simulink model "TorqueAllocator"  (R2026b)
settings: Solver=FixedStepDiscrete  StopTime=0.1  FixedStep=UnifiedControlSampleTime
settings Model: DataDictionary=VehicleData.sldd  Creator=Xu Dingyi  LastModifiedBy=29358

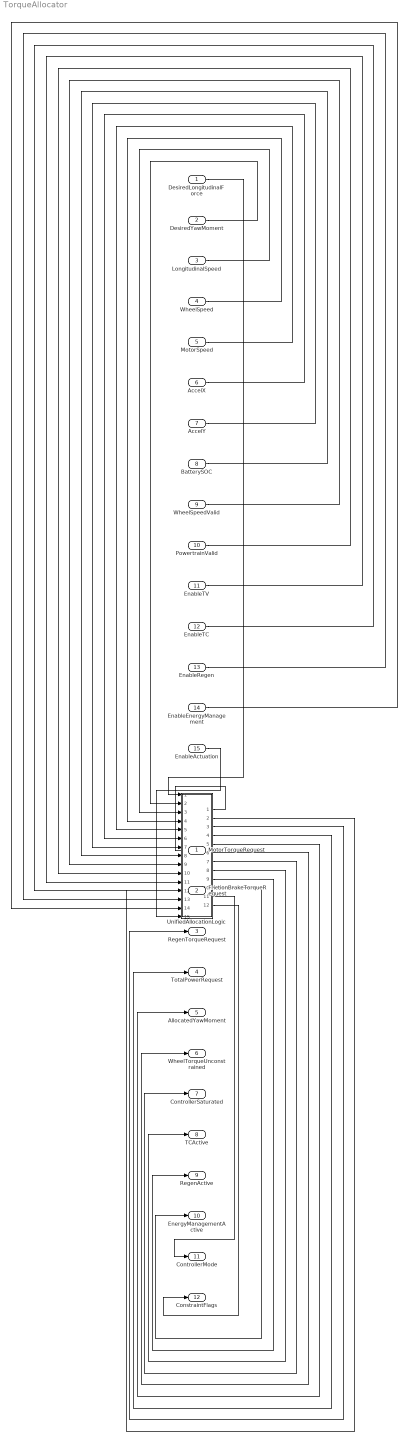
== system TorqueAllocator ==
  DesiredLongitudinalForce : Inport  OutDataTypeStr=double  PortDimensions=1
  DesiredYawMoment : Inport  Port=2  OutDataTypeStr=double  PortDimensions=1
  LongitudinalSpeed : Inport  Port=3  OutDataTypeStr=double  PortDimensions=1
  WheelSpeed : Inport  Port=4  OutDataTypeStr=double  PortDimensions=4
  MotorSpeed : Inport  Port=5  OutDataTypeStr=double  PortDimensions=4
  AccelX : Inport  Port=6  OutDataTypeStr=double  PortDimensions=1
  AccelY : Inport  Port=7  OutDataTypeStr=double  PortDimensions=1
  BatterySOC : Inport  Port=8  OutDataTypeStr=double  PortDimensions=1
  WheelSpeedValid : Inport  Port=9  OutDataTypeStr=boolean  PortDimensions=4
  PowertrainValid : Inport  Port=10  OutDataTypeStr=boolean  PortDimensions=1
  EnableTV : Inport  Port=11  OutDataTypeStr=boolean  PortDimensions=1
  EnableTC : Inport  Port=12  OutDataTypeStr=boolean  PortDimensions=1
  EnableRegen : Inport  Port=13  OutDataTypeStr=boolean  PortDimensions=1
  EnableEnergyManagement : Inport  Port=14  OutDataTypeStr=boolean  PortDimensions=1
  EnableActuation : Inport  Port=15  OutDataTypeStr=boolean  PortDimensions=1
  UnifiedAllocationLogic : Stateflow chart  TreatAsAtomicUnit=on
  MotorTorqueRequest : Outport  OutDataTypeStr=double  PortDimensions=4
  FrictionBrakeTorqueRequest : Outport  Port=2  OutDataTypeStr=double  PortDimensions=4
  RegenTorqueRequest : Outport  Port=3  OutDataTypeStr=double  PortDimensions=4
  TotalPowerRequest : Outport  Port=4  OutDataTypeStr=double  PortDimensions=1
  AllocatedYawMoment : Outport  Port=5  OutDataTypeStr=double  PortDimensions=1
  WheelTorqueUnconstrained : Outport  Port=6  OutDataTypeStr=double  PortDimensions=4
  ControllerSaturated : Outport  Port=7  OutDataTypeStr=boolean  PortDimensions=1
  TCActive : Outport  Port=8  OutDataTypeStr=boolean  PortDimensions=1
  RegenActive : Outport  Port=9  OutDataTypeStr=boolean  PortDimensions=1
  EnergyManagementActive : Outport  Port=10  OutDataTypeStr=boolean  PortDimensions=1
  ControllerMode : Outport  Port=11  OutDataTypeStr=uint8  PortDimensions=1
  ConstraintFlags : Outport  Port=12  OutDataTypeStr=uint16  PortDimensions=1
  wires:
  DesiredLongitudinalForce/1 -> UnifiedAllocationLogic/1(DesiredLongitudinalForce)
  DesiredYawMoment/1 -> UnifiedAllocationLogic/2(DesiredYawMoment)
  LongitudinalSpeed/1 -> UnifiedAllocationLogic/3(LongitudinalSpeed)
  WheelSpeed/1 -> UnifiedAllocationLogic/4(WheelSpeed)
  MotorSpeed/1 -> UnifiedAllocationLogic/5(MotorSpeed)
  AccelX/1 -> UnifiedAllocationLogic/6(AccelX)
  AccelY/1 -> UnifiedAllocationLogic/7(AccelY)
  BatterySOC/1 -> UnifiedAllocationLogic/8(BatterySOC)
  WheelSpeedValid/1 -> UnifiedAllocationLogic/9(WheelSpeedValid)
  PowertrainValid/1 -> UnifiedAllocationLogic/10(PowertrainValid)
  EnableTV/1 -> UnifiedAllocationLogic/11(EnableTV)
  EnableTC/1 -> UnifiedAllocationLogic/12(EnableTC)
  EnableRegen/1 -> UnifiedAllocationLogic/13(EnableRegen)
  EnableEnergyManagement/1 -> UnifiedAllocationLogic/14(EnableEnergyManagement)
  EnableActuation/1 -> UnifiedAllocationLogic/15(EnableActuation)
  UnifiedAllocationLogic/1(MotorTorqueRequest) -> MotorTorqueRequest/1
  UnifiedAllocationLogic/2(FrictionBrakeTorqueRequest) -> FrictionBrakeTorqueRequest/1
  UnifiedAllocationLogic/3(RegenTorqueRequest) -> RegenTorqueRequest/1
  UnifiedAllocationLogic/4(TotalPowerRequest) -> TotalPowerRequest/1
  UnifiedAllocationLogic/5(AllocatedYawMoment) -> AllocatedYawMoment/1
  UnifiedAllocationLogic/6(WheelTorqueUnconstrained) -> WheelTorqueUnconstrained/1
  UnifiedAllocationLogic/7(ControllerSaturated) -> ControllerSaturated/1
  UnifiedAllocationLogic/8(TCActive) -> TCActive/1
  UnifiedAllocationLogic/9(RegenActive) -> RegenActive/1
  UnifiedAllocationLogic/10(EnergyManagementActive) -> EnergyManagementActive/1
  UnifiedAllocationLogic/11(ControllerMode) -> ControllerMode/1
  UnifiedAllocationLogic/12(ConstraintFlags) -> ConstraintFlags/1

== stateflow chart TorqueAllocator/UnifiedAllocationLogic ==
  state Allocate
    en: PreviousMotorTorque = zeros(4,1); TCState = false(4,1);
    du: [MotorTorqueRequest, FrictionBrakeTorqueRequest, RegenTorqueRequest, TotalPowerRequest, AllocatedYawMoment, WheelTorqueUnconstrained, ControllerSaturated, TCActive, RegenActive, EnergyManagementActive, ControllerMode, ConstraintFlags, PreviousMotorTorque, TCState] = unifiedControlUnifiedAllocationStep(DesiredLongitudinalForce, DesiredYawMoment, LongitudinalSpeed, WheelSpeed, MotorSpeed, AccelX, AccelY, BatterySOC, WheelSpeedValid, PowertrainValid, EnableTV, EnableTC, EnableRegen, EnableEnergyManagement, EnableActuation, PreviousMotorTorque, TCState, UnifiedControlSampleTime, UnifiedControlVehicleMass, UnifiedControlGravity, UnifiedControlWheelbase, UnifiedControlCGHeight, UnifiedControlStaticLoadDistributionFront, UnifiedControlRollStiffnessDistributionFront, UnifiedControlTrackFront, UnifiedControlTrackRear, UnifiedControlTireEffectiveRadius, UnifiedControlLowSpeedEpsilon, UnifiedControlGearRatio, UnifiedControlGearEfficiency, UnifiedControlMotorTorqueLimit, UnifiedControlMotorSpeedLimit, UnifiedControlInverterEfficiency, UnifiedControlDrivePowerLimit, UnifiedControlRegenPowerLimit, UnifiedControlBrakeMaxTorque, UnifiedControlBatterySOCUpperLimit, UnifiedControlPowerEpsilon, UnifiedControlMotorTorqueRateLimit, UnifiedControlFrictionEstimate, UnifiedControlTCSlipOn, UnifiedControlTCSlipOff, UnifiedControlTCSlipFullCut, UnifiedControlMinimumNormalLoad, UnifiedControlEnergyDriveFraction, UnifiedControlForcePriorityWeight, UnifiedControlYawPriorityWeight, UnifiedControlRegularizationWeight, UnifiedControlAllocatorIterations);
  (default) -> Allocate
  data: DesiredLongitudinalForce input double; DesiredYawMoment input double; LongitudinalSpeed input double; WheelSpeed input double; MotorSpeed input double; AccelX input double; AccelY input double; BatterySOC input double; WheelSpeedValid input boolean; PowertrainValid input boolean; EnableTV input boolean; EnableTC input boolean; EnableRegen input boolean; EnableEnergyManagement input boolean; EnableActuation input boolean; MotorTorqueRequest output double; FrictionBrakeTorqueRequest output double; RegenTorqueRequest output double; TotalPowerRequest output double; AllocatedYawMoment output double; WheelTorqueUnconstrained output double; ControllerSaturated output boolean; TCActive output boolean; RegenActive output boolean; EnergyManagementActive output boolean; ControllerMode output uint8; ConstraintFlags output uint16; PreviousMotorTorque local double; TCState local boolean; UnifiedControlSampleTime parameter double; UnifiedControlVehicleMass parameter double; UnifiedControlGravity parameter double; UnifiedControlWheelbase parameter double; UnifiedControlCGHeight parameter double; UnifiedControlStaticLoadDistributionFront parameter double; UnifiedControlRollStiffnessDistributionFront parameter double; UnifiedControlTrackFront parameter double; UnifiedControlTrackRear parameter double; UnifiedControlTireEffectiveRadius parameter double; UnifiedControlLowSpeedEpsilon parameter double; UnifiedControlGearRatio parameter double; UnifiedControlGearEfficiency parameter double; UnifiedControlMotorTorqueLimit parameter double; UnifiedControlMotorSpeedLimit parameter double; UnifiedControlInverterEfficiency parameter double; UnifiedControlDrivePowerLimit parameter double; UnifiedControlRegenPowerLimit parameter double; UnifiedControlBrakeMaxTorque parameter double; UnifiedControlBatterySOCUpperLimit parameter double; UnifiedControlPowerEpsilon parameter double; UnifiedControlMotorTorqueRateLimit parameter double; UnifiedControlFrictionEstimate parameter double; UnifiedControlTCSlipOn parameter double; UnifiedControlTCSlipOff parameter double; UnifiedControlTCSlipFullCut parameter double; UnifiedControlMinimumNormalLoad parameter double; UnifiedControlEnergyDriveFraction parameter double; UnifiedControlForcePriorityWeight parameter double; UnifiedControlYawPriorityWeight parameter double; UnifiedControlRegularizationWeight parameter double; UnifiedControlAllocatorIterations parameter uint8
